simulink model "Controller_Simulation"  (R2025b)
settings: Solver=VariableStepAuto  StartTime=0.0  StopTime=10.0  RelTol=1e-3
values from neighbouring files (symbols this model uses):
  cg_structure = 15 + 5.353e-3    (= 15.005353)    [Final_GA.m]    (also in GA_new_new.m)
  ESC_mass_same = 40e-3    (= 0.04)    [Final_GA.m]    (also in GA_new_new.m)
  g = 9.81    [Final_GA.m]    (also in GA_new_new.m)
  m_counter = 0.15    [Final_GA.m]    (also in GA_new_new.m)
  m_struct = 35.75e-03 * 2    (= 0.0715)    [Final_GA.m]    (also in GA_new_new.m)
  mass_cable = 0.19    [Final_GA.m]    (also in GA_new_new.m)
  miu_k = 0.155    [Final_GA.m]    (also in GA_new_new.m)
  Motor_mass_small = 76e-3    (= 0.076)    [Final_GA.m]    (also in GA_new_new.m)
  prop_mass_small = 6e-3    (= 0.006)    [Final_GA.m]    (also in GA_new_new.m)
undefined symbols (not defined in the file or in its folder): DiscIntNeverNeededParam, m_cart
libraries: slpidlib x1, SignalEditorBlockLib x1
settings Model: Creator=adity  LastModifiedBy=adity

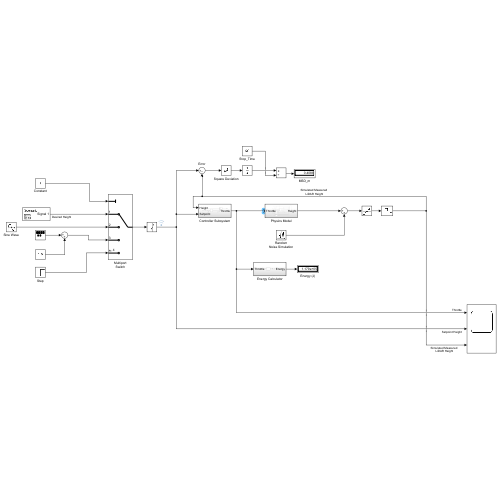
[thumbnail: Simulink's stored preview of the top-level diagram]
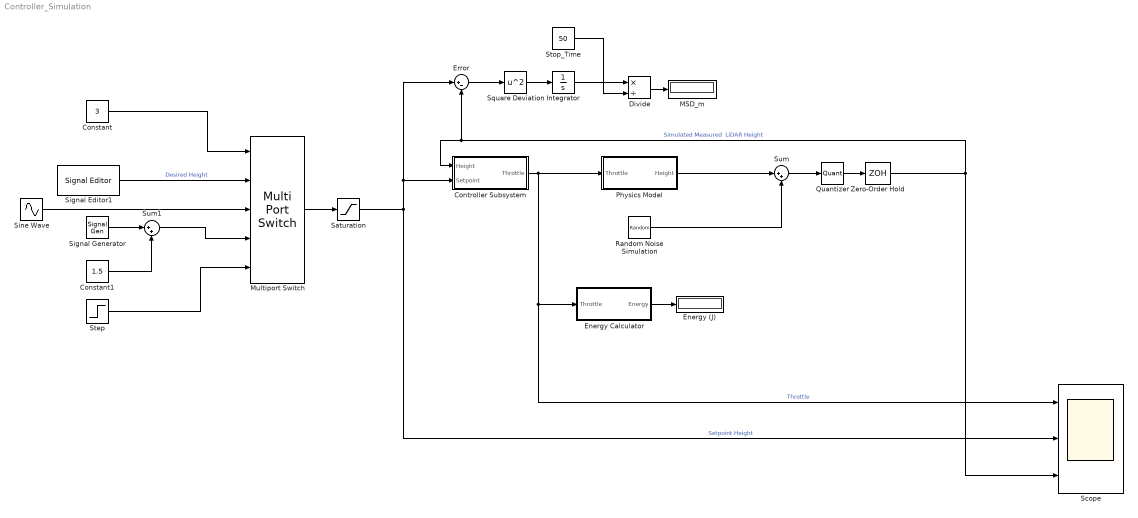
== system Controller_Simulation ==
  Constant : Constant  Value=3
  Constant1 : Constant  Value=1.5
  Controller Subsystem : Subsystem
  Divide : Product  Inputs=*/
  Energy (J) : Display
  Energy Calculator : Subsystem
  Error : Sum  Inputs=|+-
  Integrator : Integrator
  MSD_m : Display
  Multiport Switch : MultiPortSwitch  Inputs=4  SaturateOnIntegerOverflow=off  InputSameDT=off
  Physics Model : Subsystem
  Quantizer : Quantizer  QuantizationInterval=0.001
  Random Noise Simulation : RandomNumber  Variance=1e-05  SampleTime=0.05
  Saturation : Saturate  UpperLimit=3  LowerLimit=-3
  Scope : Scope  NumInputPorts=3
      settings: ActiveDisplayYMinimum=-9.1891252967878678  ActiveDisplayYMaximum=46.15249171596345
  Signal Generator : SignalGenerator  WaveForm=square  Amplitude=1.5  Units=rad/sec
  Signal Editor1 : SignalEditorBlockLib/Signal Editor  FileName=samplemission.mat  ActiveScenario=Scenario  ActiveSignal=Signal 1  IsBus=off  OutputBusObjectStr=Bus: BusObject  SampleTime=0  ZeroCross=off  OutputAfterFinalValue=Setting to zero  Unit=inherit  PreserveSignalName=on  ApplySigPropsToAllScenarios=on  ApplySigPropsToAllSignals=off  SignalPropertySource=Dialog parameters
  Sine Wave : Sin  SampleTime=0
  Square Deviation : Math  Operator=square
  Step : Step  SampleTime=0
  Stop_Time : Constant  Value=50
  Sum : Sum  Inputs=|++
  Sum1 : Sum  Inputs=|++
  Zero-Order Hold : ZeroOrderHold  SampleTime=0.05
  wires:
  Controller Subsystem/1(Throttle) -> Physics Model/1(Throttle), Energy Calculator/1(Throttle), Scope/1  "Throttle"
  Physics Model/1(Height) -> Sum/1
  Random Noise Simulation/1 -> Sum/2
  Sum/1 -> Quantizer/1
  Quantizer/1 -> Zero-Order Hold/1
  Zero-Order Hold/1 -> Scope/3, Error/2, Controller Subsystem/1(Height)  "Simulated Measured  LiDAR Height"
  Signal Editor1/1 -> Multiport Switch/2  "Desired Height"
  Signal Generator/1 -> Sum1/1
  Step/1 -> Multiport Switch/5
  Constant/1 -> Multiport Switch/1
  Multiport Switch/1 -> Saturation/1
  Saturation/1 -> Controller Subsystem/2(Setpoint), Error/1, Scope/2  "Setpoint Height"
  Energy Calculator/1(Energy) -> Energy (J)/1
  Error/1 -> Square Deviation/1
  Square Deviation/1 -> Integrator/1
  Integrator/1 -> Divide/1
  Stop_Time/1 -> Divide/2
  Divide/1 -> MSD_m/1
  Sum1/1 -> Multiport Switch/4
  Constant1/1 -> Sum1/2
  Sine Wave/1 -> Multiport Switch/3

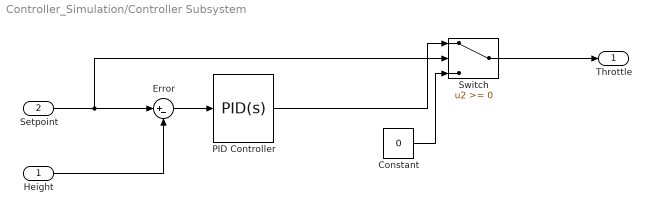
== system Controller_Simulation/Controller Subsystem ==
  Height : Inport
  Setpoint : Inport  Port=2
  Constant : Constant  Value=0
  Error : Sum  Inputs=|+-
  PID Controller : slpidlib/PID Controller  Controller=PID  Form=Parallel  TimeDomain=Continuous-time  UseExternalTs=off  SampleTime=-1  IntegratorMethod=Forward Euler  FilterMethod=Forward Euler  ControllerParametersSource=internal  P=10  I=1  UseKiTs=off  D=0  UseExternalDerivativeSource=off  N=100  UseFilter=on  TunerSelectOption=Transfer Function Based (PID Tuner App)  InitialConditionSource=internal  InitialConditionForIntegrator=0  InitialConditionForFilter=0  DifferentiatorICPrevScaledInput=0  ExternalReset=none  TrackingMode=off  Kt=1  LimitOutput=on  SatLimitsSource=internal  UpperSaturationLimit=100  LowerSaturationLimit=0  LinearizeAsGain=on  AntiWindupMode=none  Kb=1  LimitIntegrator=off  UpperIntegratorSaturationLimit=inf  LowerIntegratorSaturationLimit=-inf  POutMin=[]  POutMax=[]  IOutMin=[]  IOutMax=[]  DOutMin=[]  DOutMax=[]  NOutMin=[]  NOutMax=[]  SumOutMin=[]  SumOutMax=[]  SaturationOutMin=[]  SaturationOutMax=[]  PParamMin=[]  PParamMax=[]  IParamMin=[]  IParamMax=[]  DParamMin=[]  DParamMax=[]  NParamMin=[]  NParamMax=[]  KbParamMin=[]  KbParamMax=[]  KtParamMin=[]  KtParamMax=[]  KbOutMin=[]  KbOutMax=[]  KtOutMin=[]  KtOutMax=[]  IntegratorOutMin=[]  IntegratorOutMax=[]  FilterOutMin=[]  FilterOutMax=[]  SumI1OutMin=[]  SumI1OutMax=[]  SumI2OutMin=[]  SumI2OutMax=[]  SumI3OutMin=[]  SumI3OutMax=[]  SumI4OutMin=[]  SumI4OutMax=[]  SumDOutMin=[]  SumDOutMax=[]  DifferentiatorOutMin=[]  DifferentiatorOutMax=[]  FilterDiffOutCoefMin=[]  FilterDiffOutCoefMax=[]  ReciprocalOutMin=[]  ReciprocalOutMax=[]  SumDenOutMin=[]  SumDenOutMax=[]  SumNumOutMin=[]  SumNumOutMax=[]  DivideOutMin=[]  DivideOutMax=[]  UdiffTsProdOutMin=[]  UdiffTsProdOutMax=[]  NTsProdOutMin=[]  NTsProdOutMax=[]  UintegralTsProdOutMin=[]  UintegralTsProdOutMax=[]  UngainTsProdOutMin=[]  UngainTsProdOutMax=[]  ClampingZeroOutDataTypeStr=Inherit: Inherit via back propagation  ClampingZeroOutMin=[]  ClampingZeroOutMax=[]  FilterDenConstantOutDataTypeStr=Inherit: Inherit via back propagation  FilterDenConstantOutMin=[]  FilterDenConstantOutMax=[]  PCopyOutDataTypeStr=Inherit: Inherit via back propagation  PCopyOutMin=[]  PCopyOutMax=[]  NCopyOutDataTypeStr=Inherit: Inherit via back propagation  NCopyOutMin=[]  NCopyOutMax=[]  IntegratorContinuousStateAttributes=''  IntegratorStateMustResolveToSignalObject=off  IntegratorRTWStateStorageClass=Auto  FilterContinuousStateAttributes=''  FilterStateMustResolveToSignalObject=off  FilterRTWStateStorageClass=Auto  ParallelPVariant=InternalParameters  IdealPVariant=Disabled  IVariant=InternalParameters  DVariant=InternalParameters  IntegratorVariant=Continuous  SatVariant=Enabled  AWVariant=Passthrough  PCopyVariant=Disabled  TRVariant=Disabled  FdbkBlocksVariant=Forward  IdealPFdbkVariant=Disabled  SatFdbkVariant=Disabled  DerivativeFilterVariant=ContFilter  NVariant=InternalParameters  NCopyVariant=Disabled  FilterICVariant=InternalICsFilter  IntegratorICVariant=InternalICs  ExternalResetVariant=Disabled  TRSumVariant=Passthrough  SumFdbkVariant=Disabled  SumVariant=Sum_PID  TsampFilterVariant=InternalTs  TsampNgainVariant=Passthrough  TsampIntegralVariant=Disabled_SignalSpec  ExternalSaturationOutDataTypeStr=Inherit: Same as second input  DerivativeSourceVariant=ErrorSignal  PreIntVariant=InternalPreInt
  Switch : Switch  SaturateOnIntegerOverflow=off  InputSameDT=off
  Throttle : Outport
  wires:
  Setpoint/1 -> Switch/2, Error/1
  Height/1 -> Error/2
  Error/1 -> PID Controller/1
  PID Controller/1 -> Switch/1
  Switch/1 -> Throttle/1
  Constant/1 -> Switch/3

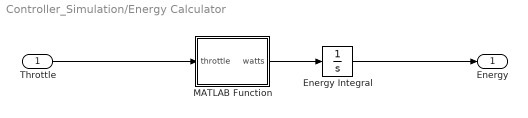
== system Controller_Simulation/Energy Calculator ==
  Throttle : Inport
  Energy Integral : Integrator
  MATLAB Function : MATLAB Function  TreatAsAtomicUnit=on
  Energy : Outport
  wires:
  Throttle/1 -> MATLAB Function/1(throttle)
  MATLAB Function/1(watts) -> Energy Integral/1
  Energy Integral/1 -> Energy/1

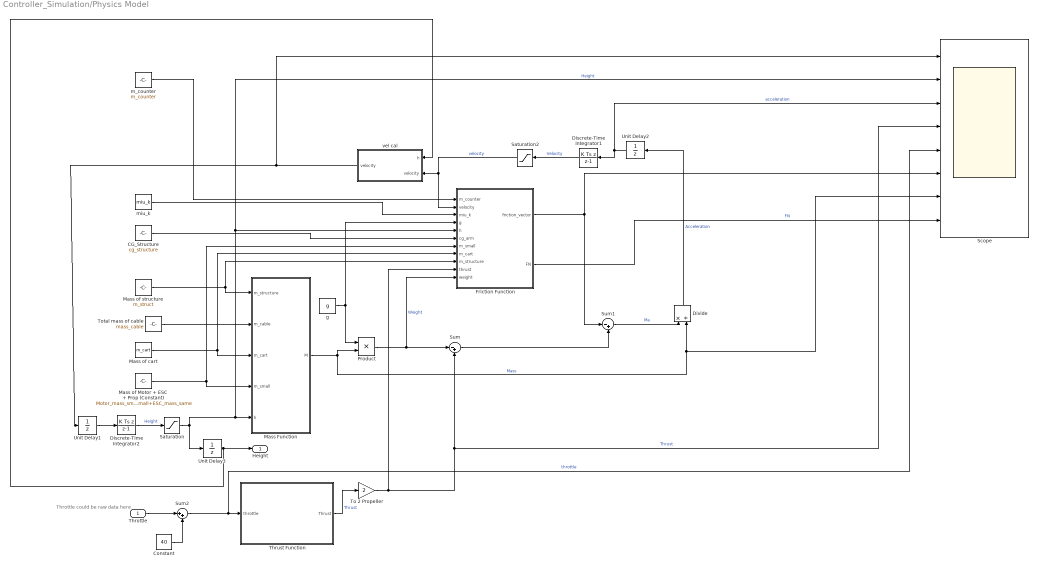
== system Controller_Simulation/Physics Model ==
  note: Throttle could be raw data here
  Throttle : Inport
  CG_Structure : Constant  Value=cg_structure
  Constant : Constant  Value=40
  Discrete-Time Integrator1 : DiscreteIntegrator  IntegratorMethod=Integration: Backward Euler  SampleTime=0.05  ICPrevOutput=DiscIntNeverNeededParam  ICPrevScaledInput=DiscIntNeverNeededParam
  Discrete-Time Integrator2 : DiscreteIntegrator  IntegratorMethod=Integration: Backward Euler  SampleTime=0.05  ICPrevOutput=DiscIntNeverNeededParam  ICPrevScaledInput=DiscIntNeverNeededParam
  Divide : Product  Inputs=*/
  Friction Function : MATLAB Function  TreatAsAtomicUnit=on
  Mass Function : MATLAB Function  TreatAsAtomicUnit=on
  Mass of Motor + ESC + Prop (Constant) : Constant  Value=Motor_mass_small+6*prop_mass_small+ESC_mass_same
  Mass of cart : Constant  Value=m_cart
  Mass of structure : Constant  Value=m_struct
  Product : Product
  Saturation : Saturate  UpperLimit=1.14  LowerLimit=0
  Saturation2 : Saturate  UpperLimit=15  LowerLimit=-15
  Scope : Scope  NumInputPorts=8
      settings: ActiveDisplayYMinimum=-1.8749999999999996  ActiveDisplayYMaximum=16.875
  Sum : Sum  Inputs=|-+
  Sum1 : Sum  Inputs=|-+
  Sum2 : Sum  Inputs=|++
  Thrust Function : MATLAB Function  TreatAsAtomicUnit=on
  To 2 Propeller : Gain  Gain=2
  Total mass of cable : Constant  Value=mass_cable
  Unit Delay1 : UnitDelay  SampleTime=0.05  HasFrameUpgradeWarning=on
  Unit Delay2 : UnitDelay  SampleTime=0.05  HasFrameUpgradeWarning=on
  Unit Delay3 : UnitDelay  SampleTime=0.05  HasFrameUpgradeWarning=on
  g : Constant  Value=g
  m_counter : Constant  Value=m_counter
  miu_k : Constant  Value=miu_k
  vel cal : MATLAB Function  TreatAsAtomicUnit=on
  Height : Outport
  wires:
  Total mass of cable/1 -> Mass Function/2(m_cable)
  Mass of Motor + ESC + Prop (Constant)/1 -> Mass Function/4(m_small), Friction Function/7(m_small)
  Discrete-Time Integrator2/1 -> Saturation/1  "Height"
  Saturation/1 -> Unit Delay3/1, Scope/2, Friction Function/5(h), Mass Function/5(h)  "Height"
  Sum1/1 -> Divide/1  "Ma"
  Friction Function/2(FN) -> Scope/8  "FN"
  Divide/1 -> Unit Delay2/1  "Acceleration"
  Mass of structure/1 -> Friction Function/9(m_structure), Mass Function/1(m_structure)
  Sum/1 -> Sum1/2
  To 2 Propeller/1 -> Scope/4, Sum/2, Friction Function/10(thrust)  "Thrust"
  Product/1 -> Sum/1, Friction Function/11(weight)  "Weight"
  Mass Function/1(M) -> Product/2, Scope/7, Divide/2  "Mass"
  miu_k/1 -> Friction Function/3(miu_k)
  g/1 -> Product/1, Friction Function/4(g)
  CG_Structure/1 -> Friction Function/6(cg_arm)
  Friction Function/1(friction_vector) -> Sum1/1, Scope/6
  Mass of cart/1 -> Mass Function/3(m_cart), Friction Function/8(m_cart)
  Unit Delay2/1 -> Discrete-Time Integrator1/1, Scope/3  "acceleration"
  Thrust Function/1(Thrust) -> To 2 Propeller/1  "Thrust"
  Discrete-Time Integrator1/1 -> Saturation2/1  "Velocity"
  Unit Delay1/1 -> Discrete-Time Integrator2/1
  Unit Delay3/1 -> Height/1, vel cal/1(h)
  Throttle/1 -> Sum2/1
  Constant/1 -> Sum2/2
  Sum2/1 -> Scope/5, Thrust Function/1(throttle)  "throttle"
  Saturation2/1 -> vel cal/2("velocity "), Friction Function/2(velocity)  "velocity"
  vel cal/1(velocity) -> Scope/1, Unit Delay1/1
  m_counter/1 -> Friction Function/1(m_counter)

== matlab function Controller_Simulation/Physics Model/Mass Function ==
  data: m_structure input; m_cable input; m_cart input; m_small input; M output; h input
function M = mass_func(m_structure,m_cable,m_cart,m_small,h)
%m_cable_calculated= 0.1958 *h^3 -0.2643 * h^2 +0.1189 *h +0.1722;
m_cable_calculated = 0.095 * h + 0.053656;
M = (2 * (m_small)) + m_cart + m_structure + m_cable_calculated;

== matlab function Controller_Simulation/Energy Calculator/MATLAB Function ==
  data: throttle input; watts output
function watts = power(throttle)

power_W = [
    1.525, 0.574, 0.574, 0.619, 0.528, 0.585, 0.593, 0.59, 0.513,...
    0.496, 4.54, 3.255, 9.484, 14.218, 19.527, 25.727, 32.509,...
    38.249, 45.079, 51.724, 56.427, 60.493, 73.286, 80.83,...
    87.083, 94.201, 100.082, 106.322, 112.106, 117.994, 123.995,...
    128.58, 133.772, 138.749, 143.756, 147.708, 151.821, 155.405,...
    158.91, 163.335, 166.856, 170.762, 174.525, 177.267, 181.534,...
    188.585, 197.784, 213.539, 223.787, 224.346, 224.563, 224.384,...
    224.196, 223.004, 223.66, 224.114, 223.565, 223.261, 223.167,...
    222.972, 223.848
];

thrust_gf = [
    4.889, 4.919, 5.269, 5.357, 5.515, 5.634, 5.801, 5.834, 5.842,...
    6.114, 6.135, 6.316, 17.075, 46.848, 75.329, 103.87, 134.015,...
    160.021, 187.923, 213.96, 236.89, 244.238, 286.999, 320.059,...
    343.454, 366.672, 389.321, 409.557, 429.939, 448.419, 469.602,...
    486.374, 502.672, 517.53, 533.561, 548.743, 561.987, 574.127,...
    587.08, 598.436, 610.385, 622.63, 634.275, 645.231, 656.905,...
    672.198, 698.929, 728.415, 771.274, 779.666, 780.836, 781.476,...
    782.351, 782.685, 782.769, 783.024, 783.137, 783.433, 783.524,...
    783.942, 784.092
];

thrust_N = thrust_gf*0.00981;

if throttle >= 0 && throttle <= 79.0425

    current_Thrust = ...
        -1.10327667e-12 * throttle^7 + ...
         3.57989341e-10 * throttle^6 + ...
        -4.57076061e-08 * throttle^5 + ...
         2.97509617e-06 * throttle^4 + ...
        -1.06350102e-04 * throttle^3 + ...
         1.98833115e-03 * throttle^2 + ...
        -3.15524313e-03 * throttle + ...
         5.50264245e-03;

elseif throttle > 79.0425 && throttle <= 100

    current_Thrust = 0.829841;

else

    error('Invalid throttle input');

end

watts = spline(thrust_N,power_W,current_Thrust);

end

== matlab function Controller_Simulation/Physics Model/Friction Function ==
  data: m_counter input; velocity input; miu_k input; g input; h input; cg_arm input; m_small input; m_cart input; m_structure input; thrust input; weight input; friction_vector output; FN output
function [friction_vector, FN] = friction_cal(m_counter, velocity, miu_k, g, h, ...
                                              cg_arm, m_small, m_cart, ...
                                              m_structure, thrust, weight)
% Total friction on a rail-mounted duocopter cart.
% Coulomb model with stiction band + active damping, applied to both
% the cart pads and the counterweight pads. Assumes 1:1 cart/counter coupling.

    % Coder-friendly init
    friction_vector         = 0;
    friction_vector_counter = 0;
    FN                      = 0;

    % Geometry & constants
    m_cable       = 0.095 * h + 0.053656;
    y_pad         = 0.171;
    y_pad_counter = y_pad;
    F_max         = 2.5506;
    F_max_counter = F_max;
    x_thrust      = cg_arm;
    cg_cart       = (7.889 + 27) * 0.001;
    cg_counter    = cg_cart;

    % Stiction band: |v| below v_eps counts as stopped; kv saturates at F_max
    v_eps = 0.001;
    kv    = F_max / v_eps;

    % Cart-side: moment balance about lower pad, abs() guards sign flip
    FN = abs( 2 * ( thrust * x_thrust ...
                    - (m_structure + 2*m_small) * g * cg_arm ...
                    - (m_cart + m_cable) * g * cg_cart ) / y_pad );

    F_dynamic       = FN * miu_k;
    resultant_force = thrust - weight;

    friction_vector = coulomb_stiction(velocity, resultant_force, ...
                                       F_dynamic, F_max, v_eps, kv);

    % Counter-side: moment from counterweight CG offset
    FN_small        = (2 * m_counter * g * cg_counter) / y_pad_counter;
    F_dynamic_small = FN_small * miu_k;
    counter_driving = m_counter * g;

    friction_vector_counter = coulomb_stiction(velocity, counter_driving, ...
                                               F_dynamic_small, F_max_counter, ...
                                               v_eps, kv);

    % Both pad sets dissipate cart KE through 1:1 coupling
    friction_vector = friction_vector + friction_vector_counter;
end


function f = coulomb_stiction(v, driving_force, F_dyn, F_max_s, v_eps, kv)
% Stick / breakaway / slide
    if abs(v) <= v_eps && abs(driving_force) < F_max_s
        f = max(min(-driving_force - kv*v, F_max_s), -F_max_s);
    elseif abs(v) <= v_eps
        f = -F_max_s * sign(driving_force);
    else
        f = -F_dyn * sign(v);
    end
end

== matlab function Controller_Simulation/Physics Model/Thrust Function ==
  data: throttle input; Thrust output
function Thrust = thrust_cal(throttle)

if throttle >= 0 && throttle <= 79.0425

    Thrust = ...
        -1.02178722e-11 * throttle^7 + ...
         3.31547781e-09 * throttle^6 + ...
        -4.23315827e-07 * throttle^5 + ...
         2.75535168e-05 * throttle^4 + ...
        -9.84949443e-04 * throttle^3 + ...
         1.84147041e-02 * throttle^2 + ...
        -2.92219275e-02 * throttle + ...
         5.09621010e-02;

elseif throttle > 79.0425 && throttle <= 100

    Thrust = 7.4300463179;

else

    error('Invalid throttle input');

end

end

== matlab function Controller_Simulation/Physics Model/vel cal ==
  data: h input; velocity input; velocity output
function velocity = vel_limit(h,velocity)
if h==0 && h== 1.44
    velocity=0;
else
    velocity=velocity;
end
